simulink model "emgCalibrationOriginal"  (R2015a)
settings: Solver=ode5  StartTime=0.0  StopTime=20  FixedStep=Ts_sim  RelTol=1e-3
undefined symbols (not defined in the file or in its folder): A_butter_acc, A_butter_cal, A_butter_low, AD622, B_butter_acc, B_butter_cal, B_butter_low, Humusoft, National_Instruments, PCI, Ts_acc, Ts_sim
libraries: sldrtlib x18, simulink x1
settings Model: Creator=Clark  LastModifiedBy=ros

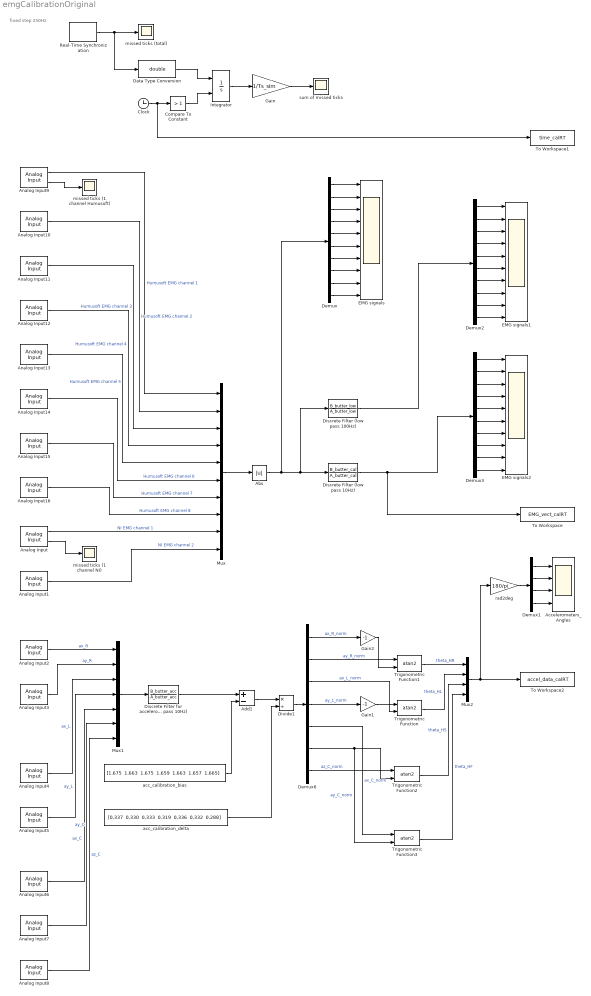
== system emgCalibrationOriginal ==
  note: fixed step 250Hz
  Abs : Abs
  Accelerometers_Angles : Scope  NumInputPorts=4
      settings: YMin=-200~-70~-200~-200  YMax=200~100~200~200  SaveName=ScopeData7
  Add1 : Sum  Inputs=+-
  Analog Input : sldrtlib/Analog Input  SampleTime=Ts_sim  MaxMissedTicks=1000  ShowMissedTicks=on  YieldWhenWaiting=off  DrvName=National_Instruments/PCI-6036E  DrvAddress=4294967295  DrvOptions=[0 0 0 0 0 0]  Channels=1  RangeMode=1  VoltRange=1  DataType=1
      settings: AttributesFormatString=National Instruments\nPCI-6036E [auto]
  Analog Input1 : sldrtlib/Analog Input  SampleTime=Ts_sim  MaxMissedTicks=1000  ShowMissedTicks=off  YieldWhenWaiting=off  DrvName=National_Instruments/PCI-6036E  DrvAddress=4294967295  DrvOptions=[0 0 0 0 0 0]  Channels=2  RangeMode=1  VoltRange=1  DataType=1
      settings: AttributesFormatString=National Instruments\nPCI-6036E [auto]
  Analog Input10 : sldrtlib/Analog Input  SampleTime=Ts_sim  MaxMissedTicks=1000  ShowMissedTicks=off  YieldWhenWaiting=off  DrvName=Humusoft/AD622  DrvAddress=4294967295  DrvOptions=zeros(1,0)  Channels=2  RangeMode=1  VoltRange=1  DataType=1
      settings: AttributesFormatString=Humusoft\nAD622 [auto]
  Analog Input11 : sldrtlib/Analog Input  SampleTime=Ts_sim  MaxMissedTicks=1000  ShowMissedTicks=off  YieldWhenWaiting=off  DrvName=Humusoft/AD622  DrvAddress=4294967295  DrvOptions=zeros(1,0)  Channels=3  RangeMode=1  VoltRange=1  DataType=1
      settings: AttributesFormatString=Humusoft\nAD622 [auto]
  Analog Input12 : sldrtlib/Analog Input  SampleTime=Ts_sim  MaxMissedTicks=1000  ShowMissedTicks=off  YieldWhenWaiting=off  DrvName=Humusoft/AD622  DrvAddress=4294967295  DrvOptions=zeros(1,0)  Channels=4  RangeMode=1  VoltRange=1  DataType=1
      settings: AttributesFormatString=Humusoft\nAD622 [auto]
  Analog Input13 : sldrtlib/Analog Input  SampleTime=Ts_sim  MaxMissedTicks=1000  ShowMissedTicks=off  YieldWhenWaiting=off  DrvName=Humusoft/AD622  DrvAddress=4294967295  DrvOptions=zeros(1,0)  Channels=5  RangeMode=1  VoltRange=1  DataType=1
      settings: AttributesFormatString=Humusoft\nAD622 [auto]
  Analog Input14 : sldrtlib/Analog Input  SampleTime=Ts_sim  MaxMissedTicks=1000  ShowMissedTicks=off  YieldWhenWaiting=off  DrvName=Humusoft/AD622  DrvAddress=4294967295  DrvOptions=zeros(1,0)  Channels=6  RangeMode=1  VoltRange=1  DataType=1
      settings: AttributesFormatString=Humusoft\nAD622 [auto]
  Analog Input15 : sldrtlib/Analog Input  SampleTime=Ts_sim  MaxMissedTicks=1000  ShowMissedTicks=off  YieldWhenWaiting=off  DrvName=Humusoft/AD622  DrvAddress=4294967295  DrvOptions=zeros(1,0)  Channels=7  RangeMode=1  VoltRange=1  DataType=1
      settings: AttributesFormatString=Humusoft\nAD622 [auto]
  Analog Input16 : sldrtlib/Analog Input  SampleTime=Ts_sim  MaxMissedTicks=1000  ShowMissedTicks=off  YieldWhenWaiting=off  DrvName=Humusoft/AD622  DrvAddress=4294967295  DrvOptions=zeros(1,0)  Channels=8  RangeMode=1  VoltRange=1  DataType=1
      settings: AttributesFormatString=Humusoft\nAD622 [auto]
  Analog Input2 : sldrtlib/Analog Input  SampleTime=Ts_acc  MaxMissedTicks=1000  ShowMissedTicks=off  YieldWhenWaiting=off  DrvName=National_Instruments/PCI-6036E  DrvAddress=4294967295  DrvOptions=[0 0 0 0 0 0]  Channels=3  RangeMode=1  VoltRange=1  DataType=1
      settings: AttributesFormatString=National Instruments\nPCI-6036E [auto]
  Analog Input3 : sldrtlib/Analog Input  SampleTime=Ts_acc  MaxMissedTicks=1000  ShowMissedTicks=off  YieldWhenWaiting=off  DrvName=National_Instruments/PCI-6036E  DrvAddress=4294967295  DrvOptions=[0 0 0 0 0 0]  Channels=4  RangeMode=1  VoltRange=1  DataType=1
      settings: AttributesFormatString=National Instruments\nPCI-6036E [auto]
  Analog Input4 : sldrtlib/Analog Input  SampleTime=Ts_acc  MaxMissedTicks=1000  ShowMissedTicks=off  YieldWhenWaiting=off  DrvName=National_Instruments/PCI-6036E  DrvAddress=4294967295  DrvOptions=[0 0 0 0 0 0]  Channels=5  RangeMode=1  VoltRange=1  DataType=1
      settings: AttributesFormatString=National Instruments\nPCI-6036E [auto]
  Analog Input5 : sldrtlib/Analog Input  SampleTime=Ts_acc  MaxMissedTicks=1000  ShowMissedTicks=off  YieldWhenWaiting=off  DrvName=National_Instruments/PCI-6036E  DrvAddress=4294967295  DrvOptions=[0 0 0 0 0 0]  Channels=6  RangeMode=1  VoltRange=1  DataType=1
      settings: AttributesFormatString=National Instruments\nPCI-6036E [auto]
  Analog Input6 : sldrtlib/Analog Input  SampleTime=Ts_acc  MaxMissedTicks=1000  ShowMissedTicks=off  YieldWhenWaiting=off  DrvName=National_Instruments/PCI-6036E  DrvAddress=4294967295  DrvOptions=[0 0 0 0 0 0]  Channels=7  RangeMode=1  VoltRange=1  DataType=1
      settings: AttributesFormatString=National Instruments\nPCI-6036E [auto]
  Analog Input7 : sldrtlib/Analog Input  SampleTime=Ts_acc  MaxMissedTicks=1000  ShowMissedTicks=off  YieldWhenWaiting=off  DrvName=National_Instruments/PCI-6036E  DrvAddress=4294967295  DrvOptions=[0 0 0 0 0 0]  Channels=8  RangeMode=1  VoltRange=1  DataType=1
      settings: AttributesFormatString=National Instruments\nPCI-6036E [auto]
  Analog Input8 : sldrtlib/Analog Input  SampleTime=Ts_acc  MaxMissedTicks=1000  ShowMissedTicks=off  YieldWhenWaiting=off  DrvName=National_Instruments/PCI-6036E  DrvAddress=4294967295  DrvOptions=[0 0 0 0 0 0]  Channels=16  RangeMode=1  VoltRange=1  DataType=1
      settings: AttributesFormatString=National Instruments\nPCI-6036E [auto]
  Analog Input9 : sldrtlib/Analog Input  SampleTime=Ts_sim  MaxMissedTicks=1000  ShowMissedTicks=on  YieldWhenWaiting=off  DrvName=Humusoft/AD622  DrvAddress=4294967295  DrvOptions=zeros(1,0)  Channels=1  RangeMode=1  VoltRange=1  DataType=1
      settings: AttributesFormatString=Humusoft\nAD622 [auto]
  Clock : Clock
  Compare To Constant : simulink/Logic and Bit Operations/Compare To Constant  relop=>  const=1  OutDataTypeStr=boolean
  Data Type Conversion : DataTypeConversion  OutDataTypeStr=double
  Demux : Demux  Outputs=10
  Demux1 : Demux
  Demux2 : Demux  Outputs=10
  Demux3 : Demux  Outputs=10
  Demux6 : Demux  Outputs=7
  Discrete Filter (low pass 100Hz) : DiscreteFilter  Numerator=B_butter_low  Denominator=A_butter_low
  Discrete Filter (low pass 10Hz) : DiscreteFilter  Numerator=B_butter_cal  Denominator=A_butter_cal
  Discrete Filter for accelerometers (low pass 10Hz) : DiscreteFilter  Numerator=B_butter_acc  Denominator=A_butter_acc
  Divide1 : Product  Inputs=*/
  EMG signals : Scope  NumInputPorts=10
      settings: TimeRange=11  YMin=0~0~0~0~0~0~0~0~2.77556e-17~0  YMax=0.75~0.4~0.3~0.15~2~2.5~0.5~0.75~0.55~0.5  SaveName=ScopeData2
  EMG signals1 : Scope  NumInputPorts=10
      settings: TimeRange=11  YMin=-0.05~-0.05~-0.05~-0.05~-0.1~-0.1~-0.2~-0.1~0.25~-0.05  YMax=0.25~0.175~0.175~0.25~0.4~0.6~0.9~0.6~0.55~0.3  SaveName=ScopeData8
  EMG signals2 : Scope  NumInputPorts=10
      settings: TimeRange=11  YMin=-0.01~-3.46945e-18~-3.46945e-18~-0.005~-3.46945e-18~-0.01~-0.005~0~0.29~0.0075  YMax=0.06~0.07~0.09~0.04~0.07~0.1~0.04~0.05~0.33~0.0225  SaveName=ScopeData6
  Gain : Gain  Gain=1/Ts_sim
  Gain1 : Gain  Gain=-1
  Gain2 : Gain  Gain=-1
  Integrator : Integrator  ExternalReset=rising
  Mux : Mux  Inputs=10
  Mux1 : Mux  Inputs=7
  Mux2 : Mux
  Real-Time Synchronization : sldrtlib/Real-Time Synchronization  SampleTime=Ts_sim  MaxMissedTicks=1000  ShowMissedTicks=on  YieldWhenWaiting=off
  To Workspace : ToWorkspace  VariableName=EMG_vect_calRT  SampleTime=-1
  To Workspace1 : ToWorkspace  VariableName=time_calRT  SampleTime=-1
  To Workspace2 : ToWorkspace  VariableName=accel_data_calRT  SaveFormat=Structure With Time  SampleTime=-1
  Trigonometric Function{,1..3} (4 alike) : Trigonometry  Operator=atan2
  acc_calibration_bias : Constant  Value="[1.675  1.663  1.675  1.659  1.663  1.657  1.665]"
  acc_calibration_delta : Constant  Value="[0.337  0.330  0.333  0.319  0.336  0.332  0.288]"
  missed ticks (1 channel Humusoft) : Scope
      settings: SaveName=ScopeData4
  missed ticks (1 channel NI) : Scope
  missed ticks (total) : Scope
  rad2deg : Gain  Gain=180/pi
  sum of missed ticks : Scope
      settings: SaveName=ScopeData3
  wires:
  Analog Input/1 -> Mux/9  "NI EMG channel 1"
  Real-Time Synchronization/1 -> Data Type Conversion/1, missed ticks (total)/1
  Analog Input/2 -> missed ticks (1 channel NI)/1
  Integrator/1 -> Gain/1
  Data Type Conversion/1 -> Integrator/1
  Gain/1 -> sum of missed ticks/1
  Clock/1 -> To Workspace1/1, Compare To Constant/1
  Compare To Constant/1 -> Integrator/2
  Analog Input1/1 -> Mux/10  "NI EMG channel 2"
  Discrete Filter (low pass 10Hz)/1 -> Demux3/1, To Workspace/1
  Mux1/1 -> Discrete Filter for accelerometers (low pass 10Hz)/1
  Demux6/3 -> Trigonometric Function/2  "ax_L_norm"
  Demux6/4 -> Gain1/1  "ay_L_norm"
  Gain1/1 -> Trigonometric Function/1
  Trigonometric Function/1 -> Mux2/2  "theta_HL"
  acc_calibration_bias/1 -> Add1/2
  Add1/1 -> Divide1/1
  acc_calibration_delta/1 -> Divide1/2
  Demux6/1 -> Gain2/1  "ax_R_norm"
  Demux6/2 -> Trigonometric Function1/1  "ay_R_norm"
  Trigonometric Function1/1 -> Mux2/1  "theta_HR"
  Divide1/1 -> Demux6/1
  Gain2/1 -> Trigonometric Function1/2
  Demux6/5 -> Trigonometric Function3/1  "ax_C_norm"
  Demux6/6 -> Trigonometric Function3/2, Trigonometric Function2/2  "ay_C_norm"
  Demux6/7 -> Trigonometric Function2/1  "az_C_norm"
  Trigonometric Function2/1 -> Mux2/3  "theta_HS"
  Trigonometric Function3/1 -> Mux2/4  "theta_HF"
  Analog Input2/1 -> Mux1/1  "ax_R"
  Analog Input3/1 -> Mux1/2  "ay_R"
  Analog Input4/1 -> Mux1/3  "ax_L"
  Analog Input5/1 -> Mux1/4  "ay_L"
  Analog Input6/1 -> Mux1/5  "ax_C"
  Analog Input7/1 -> Mux1/6  "ay_C"
  Analog Input8/1 -> Mux1/7  "az_C"
  Mux/1 -> Abs/1
  Analog Input9/2 -> missed ticks (1 channel Humusoft)/1
  Analog Input9/1 -> Mux/1  "Humusoft EMG channel 1"
  Analog Input10/1 -> Mux/2  "Humusoft EMG channel 2"
  Analog Input11/1 -> Mux/3  "Humusoft EMG channel 3"
  Analog Input12/1 -> Mux/4  "Humusoft EMG channel 4"
  Analog Input13/1 -> Mux/5  "Humusoft EMG channel 5"
  Analog Input16/1 -> Mux/8  "Humusoft EMG channel 8"
  Analog Input14/1 -> Mux/6  "Humusoft EMG channel 6"
  Analog Input15/1 -> Mux/7  "Humusoft EMG channel 7"
  Demux/1 -> EMG signals/1
  Demux/10 -> EMG signals/10
  Demux/2 -> EMG signals/2
  Demux/3 -> EMG signals/3
  Demux/4 -> EMG signals/4
  Demux/5 -> EMG signals/5
  Demux/6 -> EMG signals/6
  Demux/7 -> EMG signals/7
  Demux/8 -> EMG signals/8
  Demux/9 -> EMG signals/9
  Mux2/1 -> To Workspace2/1, rad2deg/1
  rad2deg/1 -> Demux1/1
  Demux1/1 -> Accelerometers_Angles/1
  Demux1/2 -> Accelerometers_Angles/2
  Demux1/3 -> Accelerometers_Angles/3
  Demux1/4 -> Accelerometers_Angles/4
  Discrete Filter for accelerometers (low pass 10Hz)/1 -> Add1/1
  Discrete Filter (low pass 100Hz)/1 -> Demux2/1
  Abs/1 -> Demux/1, Discrete Filter (low pass 10Hz)/1, Discrete Filter (low pass 100Hz)/1
  Demux2/1 -> EMG signals1/1
  Demux2/10 -> EMG signals1/10
  Demux2/2 -> EMG signals1/2
  Demux2/3 -> EMG signals1/3
  Demux2/4 -> EMG signals1/4
  Demux2/5 -> EMG signals1/5
  Demux2/6 -> EMG signals1/6
  Demux2/7 -> EMG signals1/7
  Demux2/8 -> EMG signals1/8
  Demux2/9 -> EMG signals1/9
  Demux3/1 -> EMG signals2/1
  Demux3/10 -> EMG signals2/10
  Demux3/2 -> EMG signals2/2
  Demux3/3 -> EMG signals2/3
  Demux3/4 -> EMG signals2/4
  Demux3/5 -> EMG signals2/5
  Demux3/6 -> EMG signals2/6
  Demux3/7 -> EMG signals2/7
  Demux3/8 -> EMG signals2/8
  Demux3/9 -> EMG signals2/9
